simulink model "2021013445李昭阳"  (R2023b)
settings: Solver=VariableStepAuto  StartTime=0.0  StopTime=10  RelTol=1e-3
libraries: sm_lib x10, nesl_utility x7, slpidlib x2
settings Model: Creator=zhaomg  LastModifiedBy=qhlzy
settings SolverCC: AlgebraicLoopSolver=TrustRegion
settings DebuggingCC: UnconnectedInputMsg=warning  UnconnectedOutputMsg=warning  UnconnectedLineMsg=warning  ArithmeticOperatorsInVariantConditions=warning
settings ModelReferenceCC: EnableRefExpFcnMdlSchedulingChecks=on
settings SFSimCC: CustomCodeUndefinedFunction=UseInterfaceOnly

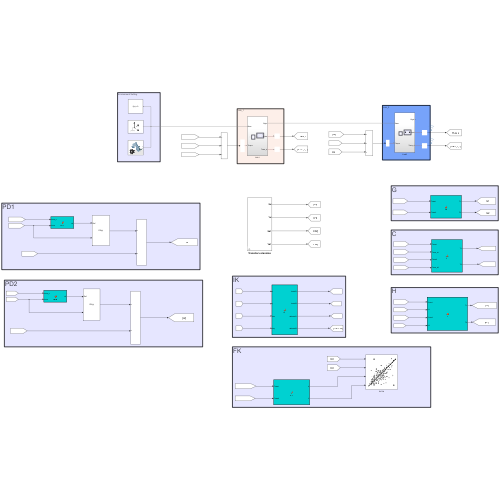
[thumbnail: Simulink's stored preview of the top-level diagram]
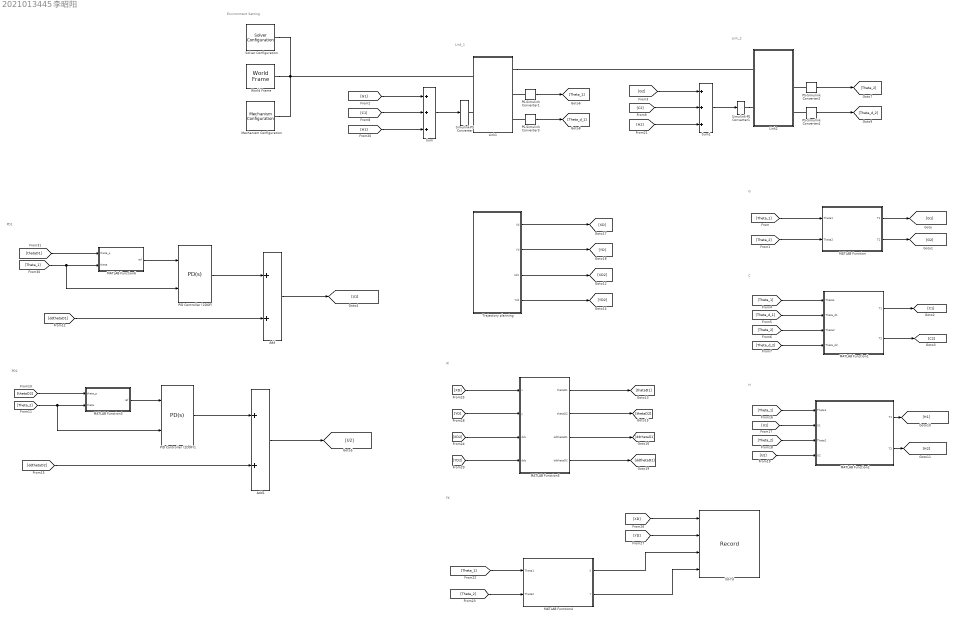
== system 2021013445李昭阳 ==
  note: PD1
  note: PD2
  note: FK
  note: H
  note: C
  note: G
  note: IK
  note: Link_2
  note: Link_1
  note: Environment Setting
  Add : Sum
  Add1 : Sum
  Link1 : Subsystem
  Link2 : Subsystem
  MATLAB Function : MATLAB Function  TreatAsAtomicUnit=on
  MATLAB Function1 : MATLAB Function  TreatAsAtomicUnit=on
  MATLAB Function2 : MATLAB Function  TreatAsAtomicUnit=on
  MATLAB Function3 : MATLAB Function  TreatAsAtomicUnit=on
  MATLAB Function4 : MATLAB Function  TreatAsAtomicUnit=on
  MATLAB Function5 : MATLAB Function  TreatAsAtomicUnit=on
  MATLAB Function6 : MATLAB Function  TreatAsAtomicUnit=on
  Mechanism Configuration : sm_lib/Utilities/Mechanism Configuration  UniformGravity=Constant  GravityVector=[0 -9.80665 0]  GravityVectorUnits=m/s^2  LinearizationDelta=0.001  JointModeTransitionNonlinearIterations=2
  PID Controller (2DOF) : slpidlib/PID Controller (2DOF)  Controller=PD  Form=Parallel  TimeDomain=Continuous-time  UseExternalTs=off  SampleTime=-1  IntegratorMethod=Forward Euler  FilterMethod=Forward Euler  ControllerParametersSource=internal  P=3396.17429419912  I=0  UseKiTs=off  D=139.457388851755  N=1053.05581536311  UseFilter=on  b=1  c=1  TunerSelectOption=Transfer Function Based (PID Tuner App)  InitialConditionSource=internal  InitialConditionForIntegrator=0  InitialConditionForFilter=0  DifferentiatorICPrevScaledInput=0  ExternalReset=none  TrackingMode=off  Kt=1  LimitOutput=off  SatLimitsSource=internal  UpperSaturationLimit=inf  LowerSaturationLimit=-inf  LinearizeAsGain=on  AntiWindupMode=none  Kb=1  LimitIntegrator=off  UpperIntegratorSaturationLimit=inf  LowerIntegratorSaturationLimit=-inf  POutMin=[]  POutMax=[]  IOutMin=[]  IOutMax=[]  DOutMin=[]  DOutMax=[]  NOutMin=[]  NOutMax=[]  bOutMin=[]  bOutMax=[]  cOutMin=[]  cOutMax=[]  SumOutMin=[]  SumOutMax=[]  SaturationOutMin=[]  SaturationOutMax=[]  PParamMin=[]  PParamMax=[]  IParamMin=[]  IParamMax=[]  DParamMin=[]  DParamMax=[]  NParamMin=[]  NParamMax=[]  bParamMin=[]  bParamMax=[]  cParamMin=[]  cParamMax=[]  KbParamMin=[]  KbParamMax=[]  KtParamMin=[]  KtParamMax=[]  KbOutMin=[]  KbOutMax=[]  KtOutMin=[]  KtOutMax=[]  IntegratorOutMin=[]  IntegratorOutMax=[]  FilterOutMin=[]  FilterOutMax=[]  SumI1OutMin=[]  SumI1OutMax=[]  SumI2OutMin=[]  SumI2OutMax=[]  SumI3OutMin=[]  SumI3OutMax=[]  SumI4OutMin=[]  SumI4OutMax=[]  SumDOutMin=[]  SumDOutMax=[]  Sum1OutMin=[]  Sum1OutMax=[]  Sum2OutMin=[]  Sum2OutMax=[]  Sum3OutMin=[]  Sum3OutMax=[]  DifferentiatorOutMin=[]  DifferentiatorOutMax=[]  FilterDiffOutCoefMin=[]  FilterDiffOutCoefMax=[]  ReciprocalOutMin=[]  ReciprocalOutMax=[]  SumDenOutMin=[]  SumDenOutMax=[]  SumNumOutMin=[]  SumNumOutMax=[]  DivideOutMin=[]  DivideOutMax=[]  UdiffTsProdOutMin=[]  UdiffTsProdOutMax=[]  NTsProdOutMin=[]  NTsProdOutMax=[]  UintegralTsProdOutMin=[]  UintegralTsProdOutMax=[]  UngainTsProdOutMin=[]  UngainTsProdOutMax=[]  ClampingZeroOutDataTypeStr=Inherit: Inherit via back propagation  ClampingZeroOutMin=[]  ClampingZeroOutMax=[]  FilterDenConstantOutDataTypeStr=Inherit: Inherit via back propagation  FilterDenConstantOutMin=[]  FilterDenConstantOutMax=[]  PCopyOutDataTypeStr=Inherit: Inherit via back propagation  PCopyOutMin=[]  PCopyOutMax=[]  NCopyOutDataTypeStr=Inherit: Inherit via back propagation  NCopyOutMin=[]  NCopyOutMax=[]  IntegratorContinuousStateAttributes=''  IntegratorStateMustResolveToSignalObject=off  IntegratorRTWStateStorageClass=Auto  FilterContinuousStateAttributes=''  FilterStateMustResolveToSignalObject=off  FilterRTWStateStorageClass=Auto  ParallelPVariant=InternalParameters  IdealPVariant=Disabled  IVariant=Disabled  DVariant=InternalParameters  bVariant=InternalParameters  cVariant=InternalParameters  IntegratorVariant=Disabled  SatVariant=Disabled  AWVariant=Disabled  PCopyVariant=Disabled  TRVariant=Disabled  FdbkBlocksVariant=Forward  IdealPFdbkVariant=Disabled  SatFdbkVariant=Disabled  DerivativeFilterVariant=ContFilter  NVariant=InternalParameters  NCopyVariant=Disabled  FilterICVariant=InternalICsFilter  IntegratorICVariant=Disabled  ExternalResetVariant=Disabled  TRSumVariant=Passthrough  SumFdbkVariant=Disabled  SumVariant=Sum_PD  TsampFilterVariant=InternalTs  TsampNgainVariant=Passthrough  TsampIntegralVariant=Disabled_SignalSpec  ExternalSaturationOutDataTypeStr=Inherit: Same as second input
  PID Controller (2DOF)1 : slpidlib/PID Controller (2DOF)  Controller=PD  Form=Parallel  TimeDomain=Continuous-time  UseExternalTs=off  SampleTime=-1  IntegratorMethod=Forward Euler  FilterMethod=Forward Euler  ControllerParametersSource=internal  P=114497.216454413  I=0  UseKiTs=off  D=531.138381467831  N=115222.186873983  UseFilter=on  b=1.0000072691455  c=0.580466499937547  TunerSelectOption=Transfer Function Based (PID Tuner App)  InitialConditionSource=internal  InitialConditionForIntegrator=0  InitialConditionForFilter=0  DifferentiatorICPrevScaledInput=0  ExternalReset=none  TrackingMode=off  Kt=1  LimitOutput=off  SatLimitsSource=internal  UpperSaturationLimit=inf  LowerSaturationLimit=-inf  LinearizeAsGain=on  AntiWindupMode=none  Kb=1  LimitIntegrator=off  UpperIntegratorSaturationLimit=inf  LowerIntegratorSaturationLimit=-inf  POutMin=[]  POutMax=[]  IOutMin=[]  IOutMax=[]  DOutMin=[]  DOutMax=[]  NOutMin=[]  NOutMax=[]  bOutMin=[]  bOutMax=[]  cOutMin=[]  cOutMax=[]  SumOutMin=[]  SumOutMax=[]  SaturationOutMin=[]  SaturationOutMax=[]  PParamMin=[]  PParamMax=[]  IParamMin=[]  IParamMax=[]  DParamMin=[]  DParamMax=[]  NParamMin=[]  NParamMax=[]  bParamMin=[]  bParamMax=[]  cParamMin=[]  cParamMax=[]  KbParamMin=[]  KbParamMax=[]  KtParamMin=[]  KtParamMax=[]  KbOutMin=[]  KbOutMax=[]  KtOutMin=[]  KtOutMax=[]  IntegratorOutMin=[]  IntegratorOutMax=[]  FilterOutMin=[]  FilterOutMax=[]  SumI1OutMin=[]  SumI1OutMax=[]  SumI2OutMin=[]  SumI2OutMax=[]  SumI3OutMin=[]  SumI3OutMax=[]  SumI4OutMin=[]  SumI4OutMax=[]  SumDOutMin=[]  SumDOutMax=[]  Sum1OutMin=[]  Sum1OutMax=[]  Sum2OutMin=[]  Sum2OutMax=[]  Sum3OutMin=[]  Sum3OutMax=[]  DifferentiatorOutMin=[]  DifferentiatorOutMax=[]  FilterDiffOutCoefMin=[]  FilterDiffOutCoefMax=[]  ReciprocalOutMin=[]  ReciprocalOutMax=[]  SumDenOutMin=[]  SumDenOutMax=[]  SumNumOutMin=[]  SumNumOutMax=[]  DivideOutMin=[]  DivideOutMax=[]  UdiffTsProdOutMin=[]  UdiffTsProdOutMax=[]  NTsProdOutMin=[]  NTsProdOutMax=[]  UintegralTsProdOutMin=[]  UintegralTsProdOutMax=[]  UngainTsProdOutMin=[]  UngainTsProdOutMax=[]  ClampingZeroOutDataTypeStr=Inherit: Inherit via back propagation  ClampingZeroOutMin=[]  ClampingZeroOutMax=[]  FilterDenConstantOutDataTypeStr=Inherit: Inherit via back propagation  FilterDenConstantOutMin=[]  FilterDenConstantOutMax=[]  PCopyOutDataTypeStr=Inherit: Inherit via back propagation  PCopyOutMin=[]  PCopyOutMax=[]  NCopyOutDataTypeStr=Inherit: Inherit via back propagation  NCopyOutMin=[]  NCopyOutMax=[]  IntegratorContinuousStateAttributes=''  IntegratorStateMustResolveToSignalObject=off  IntegratorRTWStateStorageClass=Auto  FilterContinuousStateAttributes=''  FilterStateMustResolveToSignalObject=off  FilterRTWStateStorageClass=Auto  ParallelPVariant=InternalParameters  IdealPVariant=Disabled  IVariant=Disabled  DVariant=InternalParameters  bVariant=InternalParameters  cVariant=InternalParameters  IntegratorVariant=Disabled  SatVariant=Disabled  AWVariant=Disabled  PCopyVariant=Disabled  TRVariant=Disabled  FdbkBlocksVariant=Forward  IdealPFdbkVariant=Disabled  SatFdbkVariant=Disabled  DerivativeFilterVariant=ContFilter  NVariant=InternalParameters  NCopyVariant=Disabled  FilterICVariant=InternalICsFilter  IntegratorICVariant=Disabled  ExternalResetVariant=Disabled  TRSumVariant=Passthrough  SumFdbkVariant=Disabled  SumVariant=Sum_PD  TsampFilterVariant=InternalTs  TsampNgainVariant=Passthrough  TsampIntegralVariant=Disabled_SignalSpec  ExternalSaturationOutDataTypeStr=Inherit: Same as second input
  PS-Simulink Converter1 : nesl_utility/PS-Simulink Converter  PhysicalDomain=network_engine_domain  SubClassName=ps_output  LeftPortType=input  RightPortType=output  PseudoPeriodic=off  Frequencies=[]  VectorFormat=1-D array  Unit=rad  AffineConversion=off
  PS-Simulink Converter2 : nesl_utility/PS-Simulink Converter  PhysicalDomain=network_engine_domain  SubClassName=ps_output  LeftPortType=input  RightPortType=output  PseudoPeriodic=off  Frequencies=[]  VectorFormat=1-D array  Unit=rad  AffineConversion=off
  PS-Simulink Converter3 : nesl_utility/PS-Simulink Converter  PhysicalDomain=network_engine_domain  SubClassName=ps_output  LeftPortType=input  RightPortType=output  PseudoPeriodic=off  Frequencies=[]  VectorFormat=1-D array  Unit=rad/s  AffineConversion=off
  PS-Simulink Converter4 : nesl_utility/PS-Simulink Converter  PhysicalDomain=network_engine_domain  SubClassName=ps_output  LeftPortType=input  RightPortType=output  PseudoPeriodic=off  Frequencies=[]  VectorFormat=1-D array  Unit=rad/s  AffineConversion=off
  Simulink-PS Converter : nesl_utility/Simulink-PS Converter  PhysicalDomain=network_engine_domain  SubClassName=ps_input  LeftPortType=input  RightPortType=output  PseudoPeriodic=off  Frequencies=[]  NoiseDistribution=none  NoiseParameters=[]  Unit=N*m  AffineConversion=on  FilteringAndDerivatives=provide  SimscapeFilterOrder=1  InputFilterTimeConstant=0.001  UdotUserProvided=0
  Simulink-PS Converter1 : nesl_utility/Simulink-PS Converter  PhysicalDomain=network_engine_domain  SubClassName=ps_input  LeftPortType=input  RightPortType=output  PseudoPeriodic=off  Frequencies=[]  NoiseDistribution=none  NoiseParameters=[]  Unit=N*m  AffineConversion=on  FilteringAndDerivatives=provide  SimscapeFilterOrder=1  InputFilterTimeConstant=0.001  UdotUserProvided=0
  Solver Configuration : nesl_utility/Solver Configuration  PhysicalDomain=network_engine_domain  SubClassName=solver  LeftPortType=input  RightPortType=generic  Tones=[]  Harmonics=[]  SimulateNoise=off  Profile=off  UseLocalSampling=off  EnableSwitchedLinearOptims=on  FrequencyDomain=off  UseCCode=off  RelTol=0.001  AbsTol=1e-06  MinStep=1e-09  ToWorkspace=off  RevertToSquareIcSolve=off  NumHomotopyIterations=100  PhasorMode=off  PhasorModeNumHarmonics=1  ConsistencySolver=NEWTON_FTOL  IndexReductionMethod=DerivativeReplacement  DoDC=off  ResidualTolerance=1e-12  ConsistencyTolSource=GLOBAL  ConsistencyAbsTol=0.001  ConsistencyRelTol=0.001  ConsistencyTolFactor=0.001  UseLocalSolver=off  LocalSolverChoice=NE_TRAPEZOIDAL_ADVANCER  ResolveIndetEquations=on  FunctionEvalNumThread=1  LocalSolverSampleTime=0.0001  DoFixedCost=off  MaxNonlinIter=4  MaxModeIter=2  ComputeImpulses=off  ImpulseIterations=2  LinearAlgebra=Sparse  LinearAlgebraNumThread=0  EquationFormulation=NE_TIME_EF  DelaysMemoryBudget=1024  AutomaticFiltering=on  FilteringTimeConstant=0.0001  PartitionStorageMethod=AS_NEEDED  PartitionMemoryBudget=1024  PartitionMethod=FAST  MultibodyUseLocalSolver=off  MultibodyLocalSolverChoice=ODE1  MultibodyLocalSolverSampleTime=0.001
  Sum : Sum  Inputs=+++
  Sum1 : Sum  Inputs=+++
  Trajectory planning : Subsystem  mask{x0=0.1, y0=0.1, R=0.2, T=5}
  World Frame : sm_lib/Frames and Transforms/World Frame
  Xd-Yd : Record  FileSettingsInternal="{\"entries\":[{\"content\":{\"excelSettings\":{\"content\":{},\"type\":\"Streamout.ExcelSettings\"}},\"type\":\"Streamout.FileSettingStorage\",\"uuid\":\"\"}],\"packageUris\":[\"http:\\/\\/schema.mathworks.com\\/mf0\\/streamout_blocks\\/R2020a\"],\"version\":\"1.0\"}"  Layout=[1 1]  SignalsInternal="{\"entries\":[{\"content\":{\"signals\":[{\"content\":{\"blockPath\":[],\"dimensions\":[1],\"domain\":\"\",\"lineColor\":\"#64d413\",\"plots\":[1],\"port\":1,\"sid\":[\"\"],\"signalID\":1447,\"signalName\":\"From26\"},\"type\":\"RecordBlkView.Signal\",\"uuid\":\"\"},{\"content\":{\"blockPath\":[],\"dimensions\":[1],\"domain\":\"\",\"lineColor\":\"#ff13a6\",\"plots\":[1],\"port\":2,\"sid\":[\"\"],\"signalID\":1451,\"signalName\":\"From27\"},\"type\":\"RecordBlkView.Signal\",\"uuid\":\"\"},{\"content\":{\"blockPath\":[],\"dimensions\":[1],\"domain\":\"\",\"lineColor\":\"#fe330a\",\"plots\":[1],\"port\":3,\"sid\":[\"\"],\"signalID\":1455,\"signalName\":\"MATLAB Function4:1\"},\"type\":\"RecordBlkView.Signal\",\"uuid\":\"\"},{\"content\":{\"blockPath\":[],\"dimensions\":[1],\"domain\":\"\",\"lineColor\":\"#22b573\",\"plots\":[1],\"port\":4,\"sid\":[\"\"],\"signalID\":1459,\"signalName\":\"MATLAB Function4:2\"},\"type\":\"RecordBlkView.Signal\",\"uuid\":\"\"}]},\"type\":\"RecordBlkView.InputSignals\",\"uuid\":\"\"}],\"packageUris\":[\"http:\\/\\/schema.mathworks.com\\/mf0\\/streamout_blocks\\/R2020a\"],\"version\":\"1.0\"}"  VisualizationBindings="{\"xyplotplugin\":{\"info\":[{\"series\":[{\"bindingParametersList\":[{\"parameter\":\"X-Axis\",\"signalID\":1455,\"signalName\":\"MATLAB Function4:1\"},{\"parameter\":\"Y-Axis\",\"signalID\":1459,\"signalName\":\"MATLAB Function4:2\"}],\"seriesID\":38454},{\"bindingParametersList\":[{\"parameter\":\"X-Axis\",\"signalID\":1447,\"signalName\":\"From26\"},{\"parameter\":\"Y-Axis\",\"signalID\":1451,\"signalName\":\"From27\"}],\"seriesID\":31386}],\"subplotID\":1}]}}"  CompatibilityTag=XY  st=-1
  wires:
  Sum/1 -> Simulink-PS Converter/1
  Sum1/1 -> Simulink-PS Converter1/1
  PS-Simulink Converter2/1 -> [Theta_2]
  PS-Simulink Converter3/1 -> [Theta_d_1]
  PS-Simulink Converter4/1 -> [Theta_d_2]
  PS-Simulink Converter1/1 -> [Theta_1]
  Trajectory planning/2(Yd) -> [YD]
  Trajectory planning/4(Yd1) -> [YD2]
  Trajectory planning/3(Xd1) -> [XD2]
  Trajectory planning/1(Xd) -> [XD]
  [Theta_1] -> MATLAB Function/1(Theta1)
  [Theta_2] -> MATLAB Function/2(Theta2)
  MATLAB Function/1(T1) -> [G1]
  MATLAB Function/2(T2) -> [G2]
  [Theta_d_2] -> MATLAB Function1/4(Theta_d2)
  [Theta_2] -> MATLAB Function1/3(Theta2)
  [Theta_d_1] -> MATLAB Function1/2(Theta_d1)
  [Theta_1] -> MATLAB Function1/1(Theta1)
  MATLAB Function1/1(T1) -> [C1]
  MATLAB Function1/2(T2) -> [C2]
  PID Controller (2DOF)/1 -> Add/1
  [ddthetaD1] -> Add/2
  Add/1 -> [U1]
  MATLAB Function3/1(ref) -> PID Controller (2DOF)1/1
  [Theta_2] -> PID Controller (2DOF)1/2, MATLAB Function3/2(theta)
  PID Controller (2DOF)1/1 -> Add1/1
  [ddthetaD2] -> Add1/2
  Add1/1 -> [U2]
  [Theta_1] -> MATLAB Function2/1(Theta1)
  [U1] -> MATLAB Function2/2(U1)
  [Theta_2] -> MATLAB Function2/3(Theta2)
  [U2] -> MATLAB Function2/4(U2)
  MATLAB Function2/1(T1) -> [H1]
  MATLAB Function2/2(T2) -> [H2]
  [Theta_1] -> MATLAB Function4/1(Theta1)
  [Theta_2] -> MATLAB Function4/2(Theta2)
  [XD] -> Xd-Yd/1
  [YD] -> Xd-Yd/2
  [Theta_1] -> PID Controller (2DOF)/2, MATLAB Function6/2(theta)
  MATLAB Function4/1(X) -> Xd-Yd/3
  MATLAB Function4/2(Y) -> Xd-Yd/4
  MATLAB Function6/1(ref) -> PID Controller (2DOF)/1
  [H2] -> Sum1/3
  [H1] -> Sum/3
  [XD2] -> MATLAB Function5/3(ddx)
  [XD] -> MATLAB Function5/1(x)
  [YD] -> MATLAB Function5/2(y)
  [YD2] -> MATLAB Function5/4(ddy)
  MATLAB Function5/1(thetaD1) -> [thataD1]
  MATLAB Function5/2(thetaD2) -> [thetaD2]
  MATLAB Function5/3(ddthetaD1) -> [ddthetaD1]
  MATLAB Function5/4(ddthetaD2) -> [ddthetaD2]
  [thataD1] -> MATLAB Function6/1(theta_p)
  [thetaD2] -> MATLAB Function3/1(theta_p)
  [G1] -> Sum/1
  [C1] -> Sum/2
  [G2] -> Sum1/1
  [C2] -> Sum1/2
  connections:
  World Frame/RConn1 -- Mechanism Configuration/RConn1 -- Solver Configuration/RConn1 -- Link1/LConn1
  Link1/RConn1 -- Link2/LConn1
  Simulink-PS Converter1/RConn1 -- Link2/LConn2
  PS-Simulink Converter2/LConn1 -- Link2/RConn2
  PS-Simulink Converter1/LConn1 -- Link1/RConn2
  PS-Simulink Converter3/LConn1 -- Link1/RConn3
  Simulink-PS Converter/RConn1 -- Link1/LConn2
  PS-Simulink Converter4/LConn1 -- Link2/RConn3

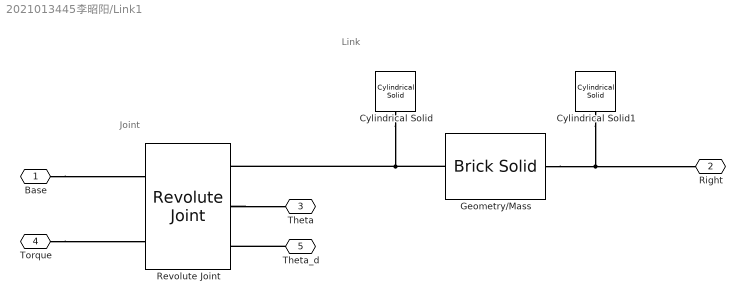
== system 2021013445李昭阳/Link1 ==
  note: Joint
  note: Link
  Cylindrical Solid : sm_lib/Body Elements/Cylindrical Solid  GraphicAmbientColor=[0.15 0.15 0.15 1.0]  BasedOnType=Density  CenterOfMass=[0 0 0]  CenterOfMassUnits=m  GraphicDiffuseColor=[1.0 0.4 0.4]  CylinderLength=2  CylinderLengthUnits=cm  CylinderRadius=2.5  CylinderRadiusUnits=cm  Density=0  DensityUnits=kg/m^3  DoExposeReferenceFrame=on  GraphicEmissiveColor=[0.0 0.0 0.0 1.0]  ExportEntireGeometry=off  SerializedFrames=<Frames/>  MarkerShape=Sphere  MarkerSize=10  GraphicType=FromGeometry  InertiaType=CalculateFromGeometry  Mass=1  MassUnits=kg  MomentsOfInertia=[1 1 1]  MomentsOfInertiaUnits=kg*m^2  GraphicOpacity=0.5  ProductsOfInertia=[0 0 0]  ProductsOfInertiaUnits=kg*m^2  GraphicShininess=75  GraphicSpecularColor=[0.5 0.5 0.5 1.0]  GraphicVisPropType=SimpleVisualProperties
  Cylindrical Solid1 : sm_lib/Body Elements/Cylindrical Solid  GraphicAmbientColor=[0.15 0.15 0.15 1.0]  BasedOnType=Density  CenterOfMass=[0 0 0]  CenterOfMassUnits=m  GraphicDiffuseColor=[1.0 0.4 0.4]  CylinderLength=2  CylinderLengthUnits=cm  CylinderRadius=2.5  CylinderRadiusUnits=cm  Density=0  DensityUnits=kg/m^3  DoExposeReferenceFrame=on  GraphicEmissiveColor=[0.0 0.0 0.0 1.0]  ExportEntireGeometry=off  SerializedFrames=<Frames/>  MarkerShape=Sphere  MarkerSize=10  GraphicType=FromGeometry  InertiaType=CalculateFromGeometry  Mass=1  MassUnits=kg  MomentsOfInertia=[1 1 1]  MomentsOfInertiaUnits=kg*m^2  GraphicOpacity=0.5  ProductsOfInertia=[0 0 0]  ProductsOfInertiaUnits=kg*m^2  GraphicShininess=75  GraphicSpecularColor=[0.5 0.5 0.5 1.0]  GraphicVisPropType=SimpleVisualProperties
  Geometry/Mass : sm_lib/Body Elements/Brick Solid  GraphicAmbientColor=[0.15 0.15 0.15 1.0]  BasedOnType=Mass  BrickDimensions=[250 50 20]  BrickDimensionsUnits=mm  CenterOfMass=[0 0 0]  CenterOfMassUnits=m  GraphicDiffuseColor=[1.0 0.4 0.4]  Density=1000  DensityUnits=kg/m^3  DoExposeReferenceFrame=off  GraphicEmissiveColor=[0.0 0.0 0.0 1.0]  ExportEntireGeometry=off  SerializedFrames=<Frames><Frame><Id>Frame1</Id><Value><Name>L</Name><Origin><Source>GeometricFeature</Source><FeatureName>-x surface</FeatureName></Origin><PrimaryAxis><DefinedDirection>+Z</DefinedDirection><Source>ReferenceFrame</Source><SourceDirection>+Z</SourceDirection><FeatureName></FeatureName></PrimaryAxis><SecondaryAxis><DefinedDirection>+X</DefinedDirection><Source>ReferenceFrame</Source><SourceDirection>+X</SourceDirection><FeatureName></FeatureName></SecondaryAxis></Value></Frame><Frame><Id>Frame2</Id><Value><Name>R</Name><Origin><Source>GeometricFeature</Source><FeatureName>+x surface</FeatureName></Origin><PrimaryAxis><DefinedDirection>+Z</DefinedDirection><Source>ReferenceFrame</Source><SourceDirection>+Z</SourceDirection><FeatureName></FeatureName></PrimaryAxis><SecondaryAxis><DefinedDirection>+X</DefinedDirection><Source>ReferenceFrame</Source><SourceDirection>+X</SourceDirection><FeatureName></FeatureName></SecondaryAxis></Value></Frame></Frames>  MarkerShape=Sphere  MarkerSize=10  GraphicType=FromGeometry  InertiaType=CalculateFromGeometry  Mass=1.0  MassUnits=kg  MomentsOfInertia=[1 1 1]  MomentsOfInertiaUnits=kg*m^2  GraphicOpacity=0.5  ProductsOfInertia=[1 1 1]  ProductsOfInertiaUnits=kg*m^2  GraphicShininess=75  GraphicSpecularColor=[0.5 0.5 0.5 1.0]  GraphicVisPropType=SimpleVisualProperties
  Revolute Joint : sm_lib/Joints/Revolute Joint  JointMode=Normal  SenseConstraintForce=off  SenseConstraintForceX=off  SenseConstraintForceY=off  SenseConstraintForceZ=off  SenseConstraintTorque=off  SenseConstraintTorqueX=off  SenseConstraintTorqueY=off  SenseConstraintTorqueZ=off  SenseTotalForce=off  SenseTotalForceX=off  SenseTotalForceY=off  SenseTotalForceZ=off  SenseTotalTorque=off  SenseTotalTorqueX=off  SenseTotalTorqueY=off  SenseTotalTorqueZ=off  CompositeWrenchDir=BaseOnFollower  CompositeWrenchFrame=FollowerFrame  EquilibriumPosition=0  EquilibriumPositionUnits=deg  SpringStiffness=0  SpringStiffnessUnits=N*m/deg  DampingCoefficient=0  DampingCoefficientUnits=N*m/(deg/s)  TorqueActuationMode=InputTorque  MotionActuationMode=ComputedMotion  SensePosition=on  SenseVelocity=on  SenseAcceleration=off  SenseTorqueForce=off  SenseLowerLimitTorqueForce=off  SenseUpperLimitTorqueForce=off  LowerLimitSpecify=off  LowerLimitBound=-90  LowerLimitBoundUnits=deg  LowerLimitStiffness=1e4  LowerLimitStiffnessUnits=N*m/deg  LowerLimitDamping=10  LowerLimitDampingUnits=N*m/(deg/s)  LowerLimitTransitionRegionWidth=0.1  LowerLimitTransitionRegionWidthUnits=deg  UpperLimitSpecify=off  UpperLimitBound=90  UpperLimitBoundUnits=deg  UpperLimitStiffness=1e4  UpperLimitStiffnessUnits=N*m/deg  UpperLimitDamping=10  UpperLimitDampingUnits=N*m/(deg/s)  UpperLimitTransitionRegionWidth=0.1  UpperLimitTransitionRegionWidthUnits=deg  PositionTargetSpecify=on  PositionTargetPriority=High  PositionTargetValue=-36  PositionTargetValueUnits=deg  VelocityTargetSpecify=off  VelocityTargetPriority=High  VelocityTargetValue=0  VelocityTargetValueUnits=deg/s
  Base : PMIOPort  Side=Left
  Right : PMIOPort  Port=2  Side=Right
  Theta : PMIOPort  Port=3  Side=Right
  Torque : PMIOPort  Port=4  Side=Left
  Theta_d : PMIOPort  Port=5  Side=Right
  connections:
  Revolute Joint/RConn2 -- Theta/RConn1
  Torque/RConn1 -- Revolute Joint/LConn2
  Geometry/Mass/RConn1 -- Right/RConn1 -- Cylindrical Solid1/RConn1
  Base/RConn1 -- Revolute Joint/LConn1
  Geometry/Mass/LConn1 -- Cylindrical Solid/RConn1 -- Revolute Joint/RConn1
  Theta_d/RConn1 -- Revolute Joint/RConn3

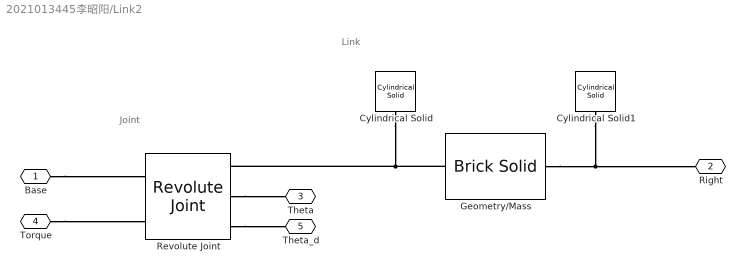
== system 2021013445李昭阳/Link2 ==
  note: Joint
  note: Link
  Cylindrical Solid : sm_lib/Body Elements/Cylindrical Solid  GraphicAmbientColor=[0.15 0.15 0.15 1.0]  BasedOnType=Density  CenterOfMass=[0 0 0]  CenterOfMassUnits=m  GraphicDiffuseColor=[1.0 0.4 0.4]  CylinderLength=2  CylinderLengthUnits=cm  CylinderRadius=2.5  CylinderRadiusUnits=cm  Density=0  DensityUnits=kg/m^3  DoExposeReferenceFrame=on  GraphicEmissiveColor=[0.0 0.0 0.0 1.0]  ExportEntireGeometry=off  SerializedFrames=<Frames/>  MarkerShape=Sphere  MarkerSize=10  GraphicType=FromGeometry  InertiaType=CalculateFromGeometry  Mass=1  MassUnits=kg  MomentsOfInertia=[1 1 1]  MomentsOfInertiaUnits=kg*m^2  GraphicOpacity=0.5  ProductsOfInertia=[0 0 0]  ProductsOfInertiaUnits=kg*m^2  GraphicShininess=75  GraphicSpecularColor=[0.5 0.5 0.5 1.0]  GraphicVisPropType=SimpleVisualProperties
  Cylindrical Solid1 : sm_lib/Body Elements/Cylindrical Solid  GraphicAmbientColor=[0.15 0.15 0.15 1.0]  BasedOnType=Density  CenterOfMass=[0 0 0]  CenterOfMassUnits=m  GraphicDiffuseColor=[0.2 0.2 1.0]  CylinderLength=2  CylinderLengthUnits=cm  CylinderRadius=2.5  CylinderRadiusUnits=cm  Density=0  DensityUnits=kg/m^3  DoExposeReferenceFrame=on  GraphicEmissiveColor=[0.0 0.0 0.0 1.0]  ExportEntireGeometry=off  SerializedFrames=<Frames/>  MarkerShape=Sphere  MarkerSize=10  GraphicType=FromGeometry  InertiaType=CalculateFromGeometry  Mass=1  MassUnits=kg  MomentsOfInertia=[1 1 1]  MomentsOfInertiaUnits=kg*m^2  GraphicOpacity=0.5  ProductsOfInertia=[0 0 0]  ProductsOfInertiaUnits=kg*m^2  GraphicShininess=75  GraphicSpecularColor=[0.5 0.5 0.5 1.0]  GraphicVisPropType=SimpleVisualProperties
  Geometry/Mass : sm_lib/Body Elements/Brick Solid  GraphicAmbientColor=[0.15 0.15 0.15 1.0]  BasedOnType=Mass  BrickDimensions=[250 50 20]  BrickDimensionsUnits=mm  CenterOfMass=[0 0 0]  CenterOfMassUnits=m  GraphicDiffuseColor=[0.2 0.4 1.0]  Density=1000  DensityUnits=kg/m^3  DoExposeReferenceFrame=off  GraphicEmissiveColor=[0.0 0.0 0.0 1.0]  ExportEntireGeometry=off  SerializedFrames=<Frames><Frame><Id>Frame1</Id><Value><Name>L</Name><Origin><Source>GeometricFeature</Source><FeatureName>-x surface</FeatureName></Origin><PrimaryAxis><DefinedDirection>+Z</DefinedDirection><Source>ReferenceFrame</Source><SourceDirection>+Z</SourceDirection><FeatureName></FeatureName></PrimaryAxis><SecondaryAxis><DefinedDirection>+X</DefinedDirection><Source>ReferenceFrame</Source><SourceDirection>+X</SourceDirection><FeatureName></FeatureName></SecondaryAxis></Value></Frame><Frame><Id>Frame2</Id><Value><Name>R</Name><Origin><Source>GeometricFeature</Source><FeatureName>+x surface</FeatureName></Origin><PrimaryAxis><DefinedDirection>+Z</DefinedDirection><Source>ReferenceFrame</Source><SourceDirection>+Z</SourceDirection><FeatureName></FeatureName></PrimaryAxis><SecondaryAxis><DefinedDirection>+X</DefinedDirection><Source>ReferenceFrame</Source><SourceDirection>+X</SourceDirection><FeatureName></FeatureName></SecondaryAxis></Value></Frame></Frames>  MarkerShape=Sphere  MarkerSize=10  GraphicType=FromGeometry  InertiaType=CalculateFromGeometry  Mass=1.0  MassUnits=kg  MomentsOfInertia=[1 1 1]  MomentsOfInertiaUnits=kg*m^2  GraphicOpacity=0.5  ProductsOfInertia=[1 1 1]  ProductsOfInertiaUnits=kg*m^2  GraphicShininess=75  GraphicSpecularColor=[0.5 0.5 0.5 1.0]  GraphicVisPropType=SimpleVisualProperties
  Revolute Joint : sm_lib/Joints/Revolute Joint  JointMode=Normal  SenseConstraintForce=off  SenseConstraintForceX=off  SenseConstraintForceY=off  SenseConstraintForceZ=off  SenseConstraintTorque=off  SenseConstraintTorqueX=off  SenseConstraintTorqueY=off  SenseConstraintTorqueZ=off  SenseTotalForce=off  SenseTotalForceX=off  SenseTotalForceY=off  SenseTotalForceZ=off  SenseTotalTorque=off  SenseTotalTorqueX=off  SenseTotalTorqueY=off  SenseTotalTorqueZ=off  CompositeWrenchDir=BaseOnFollower  CompositeWrenchFrame=FollowerFrame  EquilibriumPosition=0  EquilibriumPositionUnits=deg  SpringStiffness=0  SpringStiffnessUnits=N*m/deg  DampingCoefficient=0  DampingCoefficientUnits=N*m/(deg/s)  TorqueActuationMode=InputTorque  MotionActuationMode=ComputedMotion  SensePosition=on  SenseVelocity=on  SenseAcceleration=off  SenseTorqueForce=off  SenseLowerLimitTorqueForce=off  SenseUpperLimitTorqueForce=off  LowerLimitSpecify=off  LowerLimitBound=-90  LowerLimitBoundUnits=deg  LowerLimitStiffness=1e4  LowerLimitStiffnessUnits=N*m/deg  LowerLimitDamping=10  LowerLimitDampingUnits=N*m/(deg/s)  LowerLimitTransitionRegionWidth=0.1  LowerLimitTransitionRegionWidthUnits=deg  UpperLimitSpecify=off  UpperLimitBound=90  UpperLimitBoundUnits=deg  UpperLimitStiffness=1e4  UpperLimitStiffnessUnits=N*m/deg  UpperLimitDamping=10  UpperLimitDampingUnits=N*m/(deg/s)  UpperLimitTransitionRegionWidth=0.1  UpperLimitTransitionRegionWidthUnits=deg  PositionTargetSpecify=on  PositionTargetPriority=High  PositionTargetValue=73  PositionTargetValueUnits=deg  VelocityTargetSpecify=off  VelocityTargetPriority=High  VelocityTargetValue=0  VelocityTargetValueUnits=deg/s
  Base : PMIOPort  Side=Left
  Right : PMIOPort  Port=2  Side=Right
  Theta : PMIOPort  Port=3  Side=Right
  Torque : PMIOPort  Port=4  Side=Left
  Theta_d : PMIOPort  Port=5  Side=Right
  connections:
  Revolute Joint/RConn2 -- Theta/RConn1
  Torque/RConn1 -- Revolute Joint/LConn2
  Geometry/Mass/RConn1 -- Right/RConn1 -- Cylindrical Solid1/RConn1
  Base/RConn1 -- Revolute Joint/LConn1
  Geometry/Mass/LConn1 -- Cylindrical Solid/RConn1 -- Revolute Joint/RConn1
  Revolute Joint/RConn3 -- Theta_d/RConn1

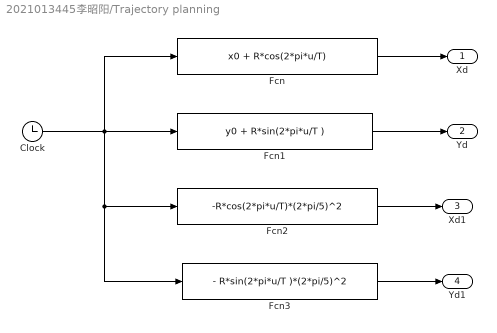
== system 2021013445李昭阳/Trajectory planning ==
  Clock : Clock
  Fcn : Fcn  Expr=x0 + R*cos(2*pi*u/T)
  Fcn1 : Fcn  Expr=y0 + R*sin(2*pi*u/T )
  Fcn2 : Fcn  Expr=-R*cos(2*pi*u/T)*(2*pi/5)^2
  Fcn3 : Fcn  Expr=- R*sin(2*pi*u/T )*(2*pi/5)^2
  Xd : Outport  VectorParamsAs1DForOutWhenUnconnected=off
  Yd : Outport  Port=2  VectorParamsAs1DForOutWhenUnconnected=off
  Xd1 : Outport  Port=3  VectorParamsAs1DForOutWhenUnconnected=off
  Yd1 : Outport  Port=4  VectorParamsAs1DForOutWhenUnconnected=off
  wires:
  Clock/1 -> Fcn/1, Fcn3/1, Fcn2/1, Fcn1/1
  Fcn/1 -> Xd/1
  Fcn1/1 -> Yd/1
  Fcn2/1 -> Xd1/1
  Fcn3/1 -> Yd1/1

== matlab function 2021013445李昭阳/MATLAB Function1 ==
  data: Theta1 input; T1 output; Theta_d1 input; Theta2 input; Theta_d2 input; T2 output
function [T1, T2] = C(Theta1, Theta_d1, Theta2, Theta_d2)

g = 9.80665;

m1 = 1.0;
L1 = 0.25;
Lc1 = 0.125;

m2 = 1.0;
L2 = 0.25;
Lc2 = 0.125;

T1 = -2 * Theta_d2 * Theta_d1 * L1 * Lc2 * m2 * sin(Theta2) - 2 * (Theta_d1 + Theta_d2) * Theta_d2 * L1 * Lc2 * m2 * sin(Theta2);
T2 = 2 * m2 * L1 * Lc2 * sin(Theta2) * Theta_d1^2;

== matlab function 2021013445李昭阳/MATLAB Function ==
  data: Theta1 input; T1 output; Theta2 input; T2 output
function [T1,T2] = G(Theta1, Theta2)

g = 9.80665;

m1 = 1.0;
L1 = 0.25;
Lc1 = 0.125;

m2 = 1.0;
L2 = 0.25;
Lc2 = 0.125;

T2 = m2 * g * Lc2 * cos(Theta1 + Theta2);
T1 = T2 + (m1 * Lc1 + m2 * L1) *cos(Theta1) * g;

== matlab function 2021013445李昭阳/MATLAB Function2 ==
  data: Theta1 input; T1 output; U1 input; Theta2 input; U2 input; T2 output
function [T1, T2] = H(Theta1, U1, Theta2, U2)

g = 9.80665;

m1 = 1.0;
L1 = 0.25;
Lc1 = 0.125;
Ic1 = 0.020833;

m2 = 1.0;
L2 = 0.25;
Lc2 = 0.125;
Ic2 = 0.020833;

T1 = (m2*L1^2 + 2*m2*cos(Theta2)*L1*Lc2 + m1*Lc1^2 + m2*Lc2^2 + Ic1 + Ic2) * U1 + (m2*Lc2^2 + L1*m2*cos(Theta2)*Lc2 + Ic2) * U2;
T2 = (m2*Lc2^2 + L1*m2*cos(Theta2)*Lc2 + Ic2) * U1 + (m2*Lc2^2 + Ic2) * U2;

== matlab function 2021013445李昭阳/MATLAB Function3 ==
  data: theta_p input; ref output; theta input
function ref = trans(theta_p, theta)
	while (theta_p - theta) >= pi
		theta_p = theta_p - 2 * pi;
	end
	while (theta_p - theta) <= -pi
		theta_p = theta_p + 2 * pi;
	end
ref = theta_p;

== matlab function 2021013445李昭阳/MATLAB Function4 ==
  data: Theta1 input; X output; Theta2 input; Y output
function [X, Y] = FK(Theta1,Theta2)

l1 = 0.25; 
l2 = 0.25;

T10 = [cos(Theta1), -sin(Theta1), 0, l1*cos(Theta1);
       sin(Theta1), cos(Theta1),  0, l1*sin(Theta1);
       0, 0, 1, 0;
       0, 0, 0, 1];

T21 = [cos(Theta2), -sin(Theta2), 0, l2*cos(Theta2);
       sin(Theta2), cos(Theta2),  0, l2*sin(Theta2);
       0, 0, 1, 0;
       0, 0, 0, 1];

T20 = T10*T21;

X = T20(1,4);
Y = T20(2,4);

== matlab function 2021013445李昭阳/MATLAB Function5 ==
  data: x input; thetaD1 output; y input; ddx input; ddy input; thetaD2 output; ddthetaD1 output; ddthetaD2 output
function [thetaD1,thetaD2,ddthetaD1,ddthetaD2] = IK(x,y,ddx,ddy)
l1 = 0.25;
l2 = 0.25;

beta = atan2(y,x);
temp = (x^2 +y^2+l1^2-l2^2)/(2*l1*sqrt(x^2+y^2));
phi = acos(temp);

thetaD1 = beta - phi;
thetaD2 = 2*phi;

J_a_inv = [-cos(thetaD1 + thetaD2)/(l1*cos(thetaD1 + thetaD2)*sin(thetaD1) - l1*sin(thetaD1 + thetaD2)*cos(thetaD1)), -sin(thetaD1 + thetaD2)/(l1*cos(thetaD1 + thetaD2)*sin(thetaD1) - l1*sin(thetaD1 + thetaD2)*cos(thetaD1));
    (l2*cos(thetaD1 + thetaD2) + l1*cos(thetaD1))/(l1*l2*cos(thetaD1 + thetaD2)*sin(thetaD1) - l1*l2*sin(thetaD1 + thetaD2)*cos(thetaD1)), (l2*sin(thetaD1 + thetaD2) + l1*sin(thetaD1))/(l1*l2*cos(thetaD1 + thetaD2)*sin(thetaD1) - l1*l2*sin(thetaD1 + thetaD2)*cos(thetaD1))];

ddthetaD1 = J_a_inv(1,:) * [ddx;ddy];
ddthetaD2 = J_a_inv(2,:) * [ddx;ddy];

== matlab function 2021013445李昭阳/MATLAB Function6 ==
  data: theta_p input; ref output; theta input
function ref = trans(theta_p, theta)
	while (theta_p - theta) >= pi
		theta_p = theta_p - 2 * pi;
	end
	while (theta_p - theta) <= -pi
		theta_p = theta_p + 2 * pi;
	end
ref = theta_p;
